simulink model "TugShield_Identification"  (R2019a)
settings: Solver=VariableStepAuto  StartTime=0.0  StopTime=10.0  RelTol=1e-3
libraries: simulink x1, TugLibrary x1
settings Model: Creator=Asus  LastModifiedBy=Asus

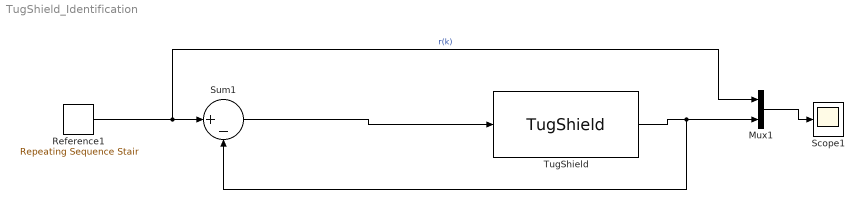
== system TugShield_Identification ==
  Mux1 : Mux  Inputs=2
  Reference1 : simulink/Sources/Repeating Sequence Stair  OutValues=[60 120 40 150 20 80 100 30].'  tsamp=5  OutMin=[]  OutMax=[]  OutDataTypeStr=double  OutputDataTypeScalingMode=double  OutDataType=fixdt(0,8)  ConRadixGroup=Best Precision: Vector-wise  OutScaling=2^-12
  Scope1 : Scope
  Sum1 : Sum  Inputs=|+-
  TugShield : TugLibrary/TugShield  OutRadio=ADC levels  Ts=0.005  CalType=Default settings (recommended)  MinVal=0  MaxVal=675
      settings: SourceProductName=AutomationShield
  wires:
  TugShield/1 -> Mux1/2, Sum1/2
  Sum1/1 -> TugShield/1
  Mux1/1 -> Scope1/1
  Reference1/1 -> Mux1/1, Sum1/1  "r(k)"
